simulink model "NDI_model"  (R2021b)
settings: Solver=ode4  StartTime=0.0  StopTime=20  FixedStep=.005  RelTol=1e-3
values from neighbouring files (symbols this model uses):
  A = [0 1; -wn^2 -2*zeta*wn]    [SetupModel.m]
  B = [0;wn^2]    [SetupModel.m]
  C = [eye(2);-wn^2 -2*zeta*wn]    [SetupModel.m]
  D = [0;0;wn^2]    [SetupModel.m]
  dist = 0    [SetupModel.m]
  I = [Ixx 0 -Ixz; 0 Iyy 0; -Ixz 0 Izz]    [NDI_quat.m]    (also in SetupModel.m = [Ixx 0 -Ixz;0 Iyy 0; -Ixz 0 Izz])
  Im = I    [SetupModel.m]
  K = lqr(A,B,Q,R,[])    [SetupModel.m]
  phi = phic(1)    [QuaternionCommand.m]    (also in SetupModel.m = 0.523598775598)
  psi = 45*pi/180    (= 0.785398163397)    [SetupModel.m]
  theta = thetac(1)    [QuaternionCommand.m]    (also in SetupModel.m = -1.0471975512)
  use_error_loop = 0    [SetupModel.m]
  x0 = [0,0,0,1,0,0,0]'    [SetupModel.m]
libraries: matrix_library x2
settings Model: Creator=17165  LastModifiedBy=17165

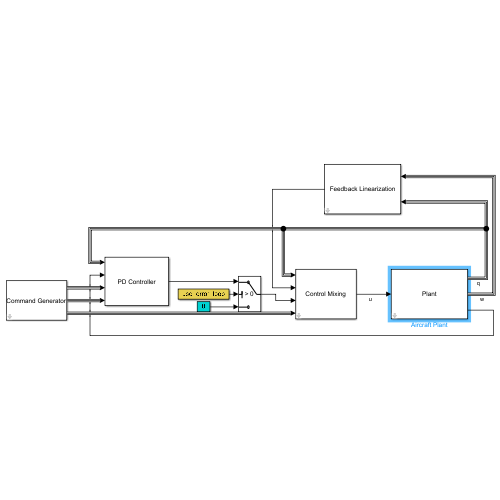
[thumbnail: Simulink's stored preview of the top-level diagram]
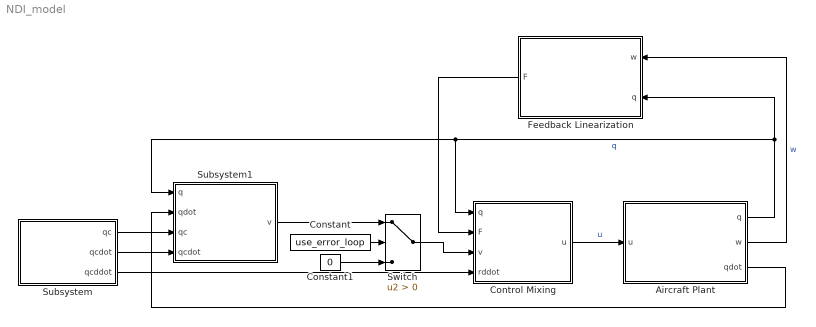
== system NDI_model ==
  Aircraft Plant : Subsystem  mask{I=I, x0=x0, dist=dist}
      mask prompts: I "Plant Moment of Inertia"; x0 "Initial Conditions"; dist "Disturbance Amplitude"
      mask Display: disp('Plant')
  Constant : Constant  Value=use_error_loop
  Constant1 : Constant  Value=0
  Control Mixing : Subsystem  mask{I=Im}
      mask prompts: I "Model Moment of Inertia"
      mask Display: disp('Control Mixing')
  Feedback Linearization : Subsystem  mask{I=Im}
      mask prompts: I "Model Moment of Inertia"
      mask Display: disp('Feedback Linearization')
  Subsystem : Subsystem  mask{A=A, B=B, C=C, D=D, phic=phi, thetac=theta, psic=psi}
      mask prompts: A "Filter A"; B "FIlter B"; C "FIlter C"; D "Filter C"; phic "Roll command"; thetac "Pitch command"; psic "Roll command"
      mask Display: disp('Command Generator')
  Subsystem1 : Subsystem
      mask Display: disp('PD Controller')
  Switch : Switch  Criteria=u2 > Threshold
  wires:
  Aircraft Plant/2(w) -> Feedback Linearization/1(w)  "w"
  Aircraft Plant/1(q) -> Feedback Linearization/2(q), Subsystem1/1(q), Control Mixing/1(q)  "q"
  Control Mixing/1(u) -> Aircraft Plant/1(u)  "u"
  Feedback Linearization/1(F) -> Control Mixing/2(F)
  Subsystem/3(qcddot) -> Control Mixing/4(rddot)
  Subsystem/1(qc) -> Subsystem1/3(qc)
  Subsystem/2(qcdot) -> Subsystem1/4(qcdot)
  Aircraft Plant/3(qdot) -> Subsystem1/2(qdot)
  Switch/1 -> Control Mixing/3(v)
  Subsystem1/1(v) -> Switch/1
  Constant/1 -> Switch/2
  Constant1/1 -> Switch/3

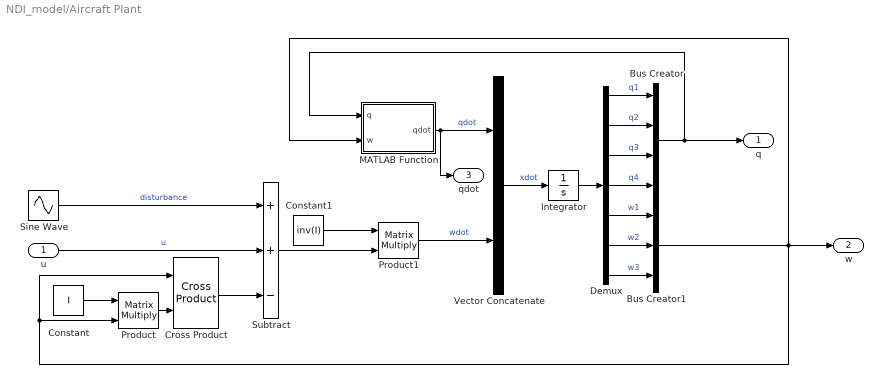
== system NDI_model/Aircraft Plant ==
  u : Inport
  Bus Creator : BusCreator  Inputs=4
  Bus Creator1 : BusCreator  Inputs=3
  Constant : Constant  Value=I
  Constant1 : Constant  Value=inv(I)
  Cross Product : matrix_library/Cross Product
      settings: SourceProductBaseCode=SL
  Demux : Demux  Outputs=7
  Integrator : Integrator  InitialCondition=x0
  MATLAB Function : MATLAB Function  TreatAsAtomicUnit=on
  Product : Product  Multiplication=Matrix(*)
  Product1 : Product  Multiplication=Matrix(*)
  Sine Wave : Sin  Amplitude=dist  SampleTime=0
  Subtract : Sum  Inputs=++-
  Vector Concatenate : Concatenate
  q : Outport
  w : Outport  Port=2
  qdot : Outport  Port=3
  wires:
  Product/1 -> Cross Product/2
  Constant/1 -> Product/1
  Subtract/1 -> Product1/2
  Constant1/1 -> Product1/1
  Product1/1 -> Vector Concatenate/2  "wdot"
  MATLAB Function/1(qdot) -> qdot/1, Vector Concatenate/1  "qdot"
  Vector Concatenate/1 -> Integrator/1  "xdot"
  Integrator/1 -> Demux/1
  Demux/1 -> Bus Creator/1  "q1"
  Demux/4 -> Bus Creator/4  "q4"
  Demux/3 -> Bus Creator/3  "q3"
  Demux/2 -> Bus Creator/2  "q2"
  Demux/5 -> Bus Creator1/1  "w1"
  Demux/6 -> Bus Creator1/2  "w2"
  Demux/7 -> Bus Creator1/3  "w3"
  Bus Creator/1 -> MATLAB Function/1(q), q/1
  Bus Creator1/1 -> w/1, MATLAB Function/2(w), Cross Product/1, Product/2
  Cross Product/1 -> Subtract/3
  u/1 -> Subtract/2  "u"
  Sine Wave/1 -> Subtract/1  "disturbance"

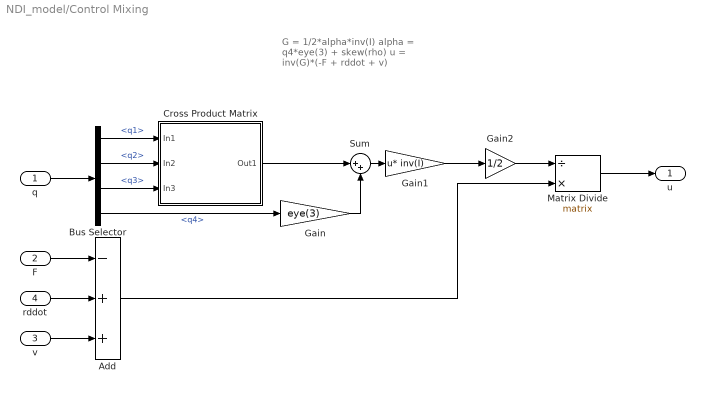
== system NDI_model/Control Mixing ==
  note: G = 1/2*alpha*inv(I)
      |
      | alpha = q4*eye(3) + skew(rho)
      |
      | u = inv(G)*(-F + rddot + v)
  q : Inport
  F : Inport  Port=2
  v : Inport  Port=3
  rddot : Inport  Port=4
  Add : Sum  Inputs=-++
  Bus Selector : BusSelector  OutputSignals=q1,q2,q3,q4
  Cross Product Matrix : Subsystem
      mask Display: disp('Cross Product Matrix')
  Gain : Gain  Gain=eye(3)
  Gain1 : Gain  Gain=inv(I)  Multiplication=Matrix(u*K)
  Gain2 : Gain  Gain=1/2
  Matrix Divide : Product  Inputs=/*  Multiplication=Matrix(*)
  Sum : Sum  Inputs=|++
  u : Outport
  wires:
  F/1 -> Add/1
  rddot/1 -> Add/2
  v/1 -> Add/3
  q/1 -> Bus Selector/1
  Bus Selector/1 -> Cross Product Matrix/1(In1)  "<q1>"
  Bus Selector/2 -> Cross Product Matrix/2(In2)  "<q2>"
  Bus Selector/3 -> Cross Product Matrix/3(In3)  "<q3>"
  Cross Product Matrix/1(Out1) -> Sum/1
  Bus Selector/4 -> Gain/1  "<q4>"
  Gain/1 -> Sum/2
  Sum/1 -> Gain1/1
  Gain1/1 -> Gain2/1
  Gain2/1 -> Matrix Divide/1
  Add/1 -> Matrix Divide/2
  Matrix Divide/1 -> u/1

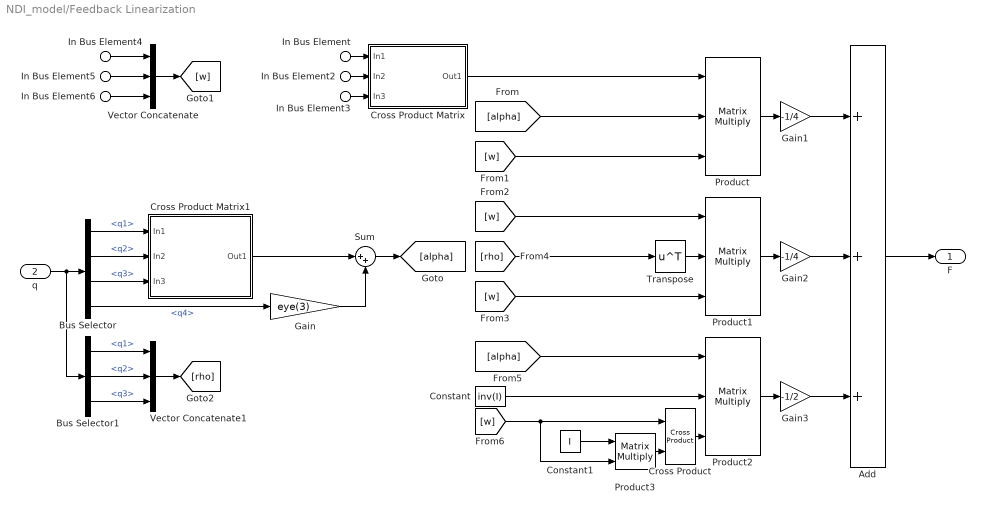
== system NDI_model/Feedback Linearization ==
  In Bus Element : Inport  PortName=w  Element=w1
  In Bus Element4 : Inport  PortName=w  Element=w1
  In Bus Element2 : Inport  PortName=w  Element=w2
  In Bus Element5 : Inport  PortName=w  Element=w2
  In Bus Element3 : Inport  PortName=w  Element=w3
  In Bus Element6 : Inport  PortName=w  Element=w3
  q : Inport  Port=2
  Add : Sum  Inputs=+++
  Bus Selector : BusSelector  OutputSignals=q1,q2,q3,q4
  Bus Selector1 : BusSelector  OutputSignals=q1,q2,q3
  Constant : Constant  Value=inv(I)
  Constant1 : Constant  Value=I
  Cross Product : matrix_library/Cross Product
      settings: SourceProductBaseCode=SL
  Cross Product Matrix : Subsystem
      mask Display: disp('Cross Product Matrix')
  Cross Product Matrix1 : Subsystem
      mask Display: disp('Cross Product Matrix')
  Gain : Gain  Gain=eye(3)
  Gain1 : Gain  Gain=-1/4
  Gain2 : Gain  Gain=-1/4
  Gain3 : Gain  Gain=-1/2
  Product : Product  Inputs=3  Multiplication=Matrix(*)
  Product1 : Product  Inputs=3  Multiplication=Matrix(*)
  Product2 : Product  Inputs=3  Multiplication=Matrix(*)
  Product3 : Product  Multiplication=Matrix(*)
  Sum : Sum  Inputs=|++
  Transpose : Math  Operator=transpose  SaturateOnIntegerOverflow=on
  Vector Concatenate : Concatenate  NumInputs=3
  Vector Concatenate1 : Concatenate  NumInputs=3
  F : Outport
  wires:
  In Bus Element/1 -> Cross Product Matrix/1(In1)
  In Bus Element2/1 -> Cross Product Matrix/2(In2)
  In Bus Element3/1 -> Cross Product Matrix/3(In3)
  In Bus Element5/1 -> Vector Concatenate/2
  In Bus Element4/1 -> Vector Concatenate/1
  In Bus Element6/1 -> Vector Concatenate/3
  Gain/1 -> Sum/2
  Bus Selector/1 -> Cross Product Matrix1/1(In1)  "<q1>"
  Bus Selector/2 -> Cross Product Matrix1/2(In2)  "<q2>"
  q/1 -> Bus Selector1/1, Bus Selector/1
  Cross Product Matrix1/1(Out1) -> Sum/1
  Bus Selector/4 -> Gain/1  "<q4>"
  Bus Selector/3 -> Cross Product Matrix1/3(In3)  "<q3>"
  Sum/1 -> [alpha]
  Cross Product Matrix/1(Out1) -> Product/1
  [alpha] -> Product/2
  Vector Concatenate/1 -> [w]
  [w] -> Product/3
  Bus Selector1/3 -> Vector Concatenate1/3  "<q3>"
  Bus Selector1/1 -> Vector Concatenate1/1  "<q1>"
  Bus Selector1/2 -> Vector Concatenate1/2  "<q2>"
  Vector Concatenate1/1 -> [rho]
  Product/1 -> Gain1/1
  [w] -> Product1/1
  [w] -> Product1/3
  Transpose/1 -> Product1/2
  [rho] -> Transpose/1
  Product1/1 -> Gain2/1
  [alpha] -> Product2/1
  Constant/1 -> Product2/2
  Constant1/1 -> Product3/1
  Product3/1 -> Cross Product/2
  Cross Product/1 -> Product2/3
  [w] -> Product3/2, Cross Product/1
  Product2/1 -> Gain3/1
  Gain2/1 -> Add/2
  Gain1/1 -> Add/1
  Gain3/1 -> Add/3
  Add/1 -> F/1

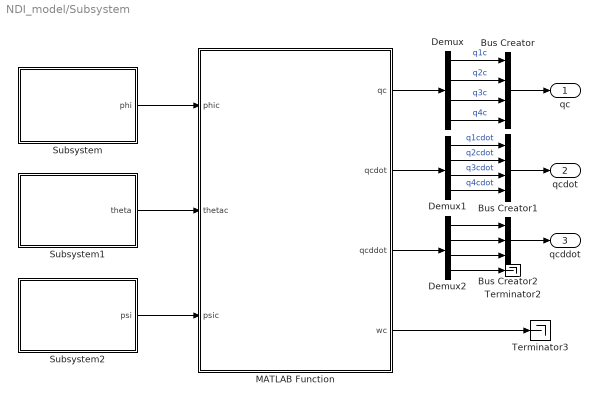
== system NDI_model/Subsystem ==
  Bus Creator : BusCreator  Inputs=4
  Bus Creator1 : BusCreator  Inputs=4
  Bus Creator2 : BusCreator  Inputs=3
  Demux : Demux
  Demux1 : Demux
  Demux2 : Demux
  MATLAB Function : MATLAB Function  TreatAsAtomicUnit=on
  Subsystem : Subsystem  mask{A=A, B=B, C=C, D=D, amp=phic}
      mask prompts: A "FIlter A Matrix"; B "Filter B Matrix"; C "Filter C Matrix"; D "Filter D Matrix"; amp "Quaternion Command"
      mask Display: disp('Filtered Command')
  Subsystem1 : Subsystem  mask{A=A, B=B, C=C, D=D, amp=thetac}
      mask prompts: A "FIlter A Matrix"; B "Filter B Matrix"; C "Filter C Matrix"; D "Filter D Matrix"; amp "Quaternion Command"
      mask Display: disp('Filtered Command')
  Subsystem2 : Subsystem  mask{A=A, B=B, C=C, D=D, amp=psic}
      mask prompts: A "FIlter A Matrix"; B "Filter B Matrix"; C "Filter C Matrix"; D "Filter D Matrix"; amp "Quaternion Command"
      mask Display: disp('Filtered Command')
  Terminator2 : Terminator
  Terminator3 : Terminator
  qc : Outport
  qcdot : Outport  Port=2
  qcddot : Outport  Port=3
  wires:
  Subsystem/1(phi) -> MATLAB Function/1(phic)
  Subsystem1/1(theta) -> MATLAB Function/2(thetac)
  Subsystem2/1(psi) -> MATLAB Function/3(psic)
  MATLAB Function/2(qcdot) -> Demux1/1
  MATLAB Function/1(qc) -> Demux/1
  MATLAB Function/4(wc) -> Terminator3/1
  Demux/4 -> Bus Creator/4  "q4c"
  Bus Creator/1 -> qc/1
  Demux1/2 -> Bus Creator1/2  "q2cdot"
  Bus Creator1/1 -> qcdot/1
  Demux1/1 -> Bus Creator1/1  "q1cdot"
  Demux1/3 -> Bus Creator1/3  "q3cdot"
  Demux1/4 -> Bus Creator1/4  "q4cdot"
  Bus Creator2/1 -> qcddot/1
  MATLAB Function/3(qcddot) -> Demux2/1
  Demux2/1 -> Bus Creator2/1
  Demux2/2 -> Bus Creator2/2
  Demux2/3 -> Bus Creator2/3
  Demux2/4 -> Terminator2/1
  Demux/1 -> Bus Creator/1  "q1c"
  Demux/2 -> Bus Creator/2  "q2c"
  Demux/3 -> Bus Creator/3  "q3c"

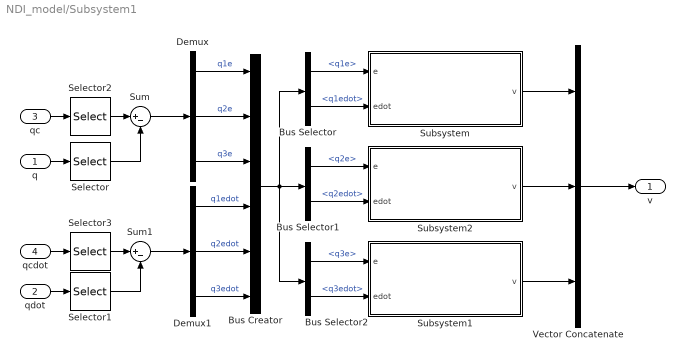
== system NDI_model/Subsystem1 ==
  q : Inport
  qdot : Inport  Port=2
  qc : Inport  Port=3
  qcdot : Inport  Port=4
  Bus Creator : BusCreator  Inputs=6
  Bus Selector : BusSelector  OutputSignals=q1e,q1edot
  Bus Selector1 : BusSelector  OutputSignals=q2e,q2edot
  Bus Selector2 : BusSelector  OutputSignals=q3e,q3edot
  Demux : Demux  Outputs=3
  Demux1 : Demux  Outputs=3
  Selector{,1..3} (4 alike) : Selector  InputPortWidth=4  IndexOptions=Index vector (dialog)  Indices=[1 2 3]  OutputSizes=1
  Subsystem : Subsystem  mask{Kp=K(1), Kd=K(2)}
      mask Display: disp('PD-Compensator')
  Subsystem1 : Subsystem  mask{Kp=K(1), Kd=K(2)}
      mask Display: disp('PD-Compensator')
  Subsystem2 : Subsystem  mask{Kp=K(1), Kd=K(2)}
      mask Display: disp('PD-Compensator')
  Sum : Sum  Inputs=|+-
  Sum1 : Sum  Inputs=|+-
  Vector Concatenate : Concatenate  NumInputs=3
  v : Outport
  wires:
  Vector Concatenate/1 -> v/1
  Subsystem/1(v) -> Vector Concatenate/1
  Subsystem2/1(v) -> Vector Concatenate/2
  Subsystem1/1(v) -> Vector Concatenate/3
  Sum/1 -> Demux/1
  Sum1/1 -> Demux1/1
  Demux/1 -> Bus Creator/1  "q1e"
  Demux/2 -> Bus Creator/2  "q2e"
  Demux/3 -> Bus Creator/3  "q3e"
  Demux1/1 -> Bus Creator/4  "q1edot"
  Demux1/2 -> Bus Creator/5  "q2edot"
  Demux1/3 -> Bus Creator/6  "q3edot"
  Bus Selector/1 -> Subsystem/1(e)  "<q1e>"
  Bus Selector/2 -> Subsystem/2(edot)  "<q1edot>"
  Bus Selector2/2 -> Subsystem1/2(edot)  "<q3edot>"
  Bus Selector2/1 -> Subsystem1/1(e)  "<q3e>"
  Bus Selector1/1 -> Subsystem2/1(e)  "<q2e>"
  Bus Selector1/2 -> Subsystem2/2(edot)  "<q2edot>"
  Bus Creator/1 -> Bus Selector2/1, Bus Selector/1, Bus Selector1/1
  q/1 -> Selector/1
  Selector/1 -> Sum/2
  qdot/1 -> Selector1/1
  Selector1/1 -> Sum1/2
  qc/1 -> Selector2/1
  Selector2/1 -> Sum/1
  qcdot/1 -> Selector3/1
  Selector3/1 -> Sum1/1

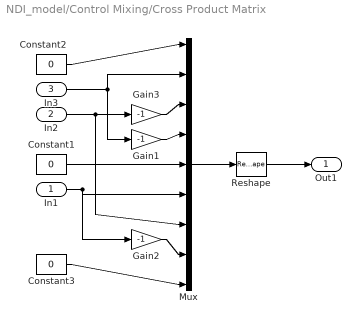
== system NDI_model/Control Mixing/Cross Product Matrix ==
  In1 : Inport
  In2 : Inport  Port=2
  In3 : Inport  Port=3
  Constant1 : Constant  Value=0
  Constant2 : Constant  Value=0
  Constant3 : Constant  Value=0
  Gain1 : Gain  Gain=-1
  Gain2 : Gain  Gain=-1
  Gain3 : Gain  Gain=-1
  Mux : Mux  Inputs=9
  Reshape : Reshape  OutputDimensionality=Customize  OutputDimensions=[3,3]
  Out1 : Outport
  wires:
  Constant2/1 -> Mux/1
  Constant1/1 -> Mux/5
  In1/1 -> Gain2/1, Mux/6
  In3/1 -> Gain1/1, Mux/2
  Constant3/1 -> Mux/9
  Reshape/1 -> Out1/1
  Mux/1 -> Reshape/1
  Gain3/1 -> Mux/3
  In2/1 -> Mux/7, Gain3/1
  Gain1/1 -> Mux/4
  Gain2/1 -> Mux/8

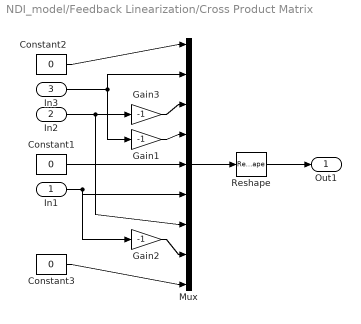
== system NDI_model/Feedback Linearization/Cross Product Matrix ==
  In1 : Inport
  In2 : Inport  Port=2
  In3 : Inport  Port=3
  Constant1 : Constant  Value=0
  Constant2 : Constant  Value=0
  Constant3 : Constant  Value=0
  Gain1 : Gain  Gain=-1
  Gain2 : Gain  Gain=-1
  Gain3 : Gain  Gain=-1
  Mux : Mux  Inputs=9
  Reshape : Reshape  OutputDimensionality=Customize  OutputDimensions=[3,3]
  Out1 : Outport
  wires:
  Constant2/1 -> Mux/1
  Constant1/1 -> Mux/5
  In1/1 -> Gain2/1, Mux/6
  In3/1 -> Gain1/1, Mux/2
  Constant3/1 -> Mux/9
  Reshape/1 -> Out1/1
  Mux/1 -> Reshape/1
  Gain3/1 -> Mux/3
  In2/1 -> Mux/7, Gain3/1
  Gain1/1 -> Mux/4
  Gain2/1 -> Mux/8

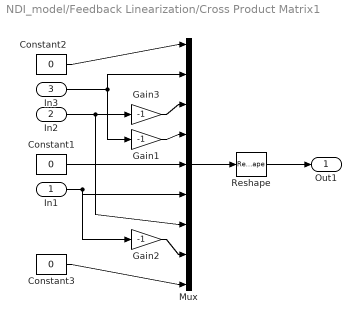
== system NDI_model/Feedback Linearization/Cross Product Matrix1 ==
  In1 : Inport
  In2 : Inport  Port=2
  In3 : Inport  Port=3
  Constant1 : Constant  Value=0
  Constant2 : Constant  Value=0
  Constant3 : Constant  Value=0
  Gain1 : Gain  Gain=-1
  Gain2 : Gain  Gain=-1
  Gain3 : Gain  Gain=-1
  Mux : Mux  Inputs=9
  Reshape : Reshape  OutputDimensionality=Customize  OutputDimensions=[3,3]
  Out1 : Outport
  wires:
  Constant2/1 -> Mux/1
  Constant1/1 -> Mux/5
  In1/1 -> Gain2/1, Mux/6
  In3/1 -> Gain1/1, Mux/2
  Constant3/1 -> Mux/9
  Reshape/1 -> Out1/1
  Mux/1 -> Reshape/1
  Gain3/1 -> Mux/3
  In2/1 -> Mux/7, Gain3/1
  Gain1/1 -> Mux/4
  Gain2/1 -> Mux/8

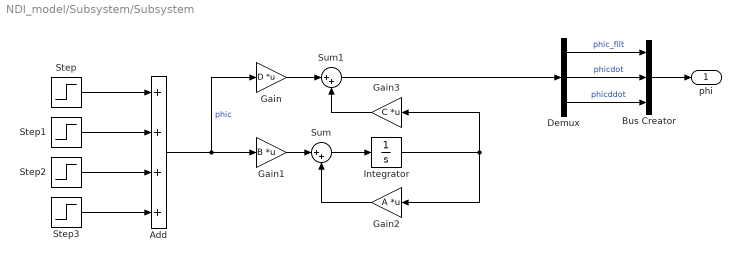
== system NDI_model/Subsystem/Subsystem ==
  Add : Sum  Inputs=++++
  Bus Creator : BusCreator  Inputs=3
  Demux : Demux  Outputs=3
  Gain : Gain  Gain=D  Multiplication=Matrix(K*u)
  Gain1 : Gain  Gain=B  Multiplication=Matrix(K*u)
  Gain2 : Gain  Gain=A  Multiplication=Matrix(K*u)
  Gain3 : Gain  Gain=C  Multiplication=Matrix(K*u)
  Integrator : Integrator
  Step : Step  After=amp  SampleTime=0
  Step1 : Step  Time=6  After=-amp  SampleTime=0
  Step2 : Step  Time=6  After=-amp  SampleTime=0
  Step3 : Step  Time=11  After=amp  SampleTime=0
  Sum : Sum  Inputs=|++
  Sum1 : Sum  Inputs=|++
  phi : Outport
  wires:
  Gain/1 -> Sum1/1
  Sum1/1 -> Demux/1
  Add/1 -> Gain/1, Gain1/1  "phic"
  Step2/1 -> Add/3
  Gain1/1 -> Sum/1
  Integrator/1 -> Gain2/1, Gain3/1
  Step1/1 -> Add/2
  Step/1 -> Add/1
  Gain3/1 -> Sum1/2
  Step3/1 -> Add/4
  Gain2/1 -> Sum/2
  Sum/1 -> Integrator/1
  Bus Creator/1 -> phi/1
  Demux/1 -> Bus Creator/1  "phic_filt"
  Demux/2 -> Bus Creator/2  "phicdot"
  Demux/3 -> Bus Creator/3  "phicddot"

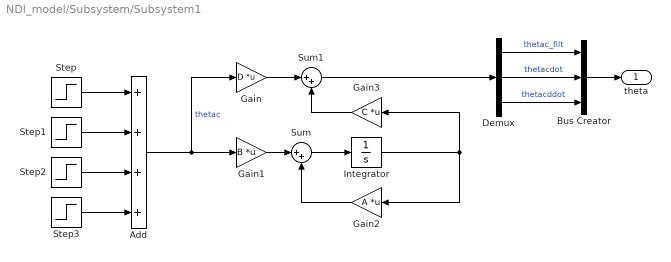
== system NDI_model/Subsystem/Subsystem1 ==
  Add : Sum  Inputs=++++
  Bus Creator : BusCreator  Inputs=3
  Demux : Demux  Outputs=3
  Gain : Gain  Gain=D  Multiplication=Matrix(K*u)
  Gain1 : Gain  Gain=B  Multiplication=Matrix(K*u)
  Gain2 : Gain  Gain=A  Multiplication=Matrix(K*u)
  Gain3 : Gain  Gain=C  Multiplication=Matrix(K*u)
  Integrator : Integrator
  Step : Step  After=amp  SampleTime=0
  Step1 : Step  Time=6  After=-amp  SampleTime=0
  Step2 : Step  Time=6  After=-amp  SampleTime=0
  Step3 : Step  Time=11  After=amp  SampleTime=0
  Sum : Sum  Inputs=|++
  Sum1 : Sum  Inputs=|++
  theta : Outport
  wires:
  Gain/1 -> Sum1/1
  Add/1 -> Gain/1, Gain1/1  "thetac"
  Step2/1 -> Add/3
  Gain1/1 -> Sum/1
  Integrator/1 -> Gain2/1, Gain3/1
  Step1/1 -> Add/2
  Step/1 -> Add/1
  Gain3/1 -> Sum1/2
  Step3/1 -> Add/4
  Gain2/1 -> Sum/2
  Sum/1 -> Integrator/1
  Demux/3 -> Bus Creator/3  "thetacddot"
  Demux/1 -> Bus Creator/1  "thetac_filt"
  Sum1/1 -> Demux/1
  Bus Creator/1 -> theta/1
  Demux/2 -> Bus Creator/2  "thetacdot"

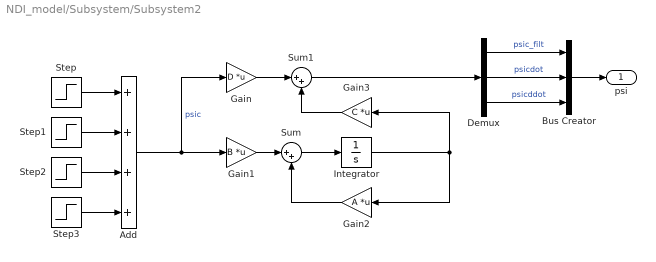
== system NDI_model/Subsystem/Subsystem2 ==
  Add : Sum  Inputs=++++
  Bus Creator : BusCreator  Inputs=3
  Demux : Demux  Outputs=3
  Gain : Gain  Gain=D  Multiplication=Matrix(K*u)
  Gain1 : Gain  Gain=B  Multiplication=Matrix(K*u)
  Gain2 : Gain  Gain=A  Multiplication=Matrix(K*u)
  Gain3 : Gain  Gain=C  Multiplication=Matrix(K*u)
  Integrator : Integrator
  Step : Step  After=amp  SampleTime=0
  Step1 : Step  Time=6  After=-amp  SampleTime=0
  Step2 : Step  Time=6  After=-amp  SampleTime=0
  Step3 : Step  Time=11  After=amp  SampleTime=0
  Sum : Sum  Inputs=|++
  Sum1 : Sum  Inputs=|++
  psi : Outport
  wires:
  Gain/1 -> Sum1/1
  Add/1 -> Gain/1, Gain1/1  "psic"
  Step2/1 -> Add/3
  Gain1/1 -> Sum/1
  Integrator/1 -> Gain2/1, Gain3/1
  Step1/1 -> Add/2
  Step/1 -> Add/1
  Gain3/1 -> Sum1/2
  Step3/1 -> Add/4
  Gain2/1 -> Sum/2
  Sum/1 -> Integrator/1
  Demux/3 -> Bus Creator/3  "psicddot"
  Demux/1 -> Bus Creator/1  "psic_filt"
  Sum1/1 -> Demux/1
  Bus Creator/1 -> psi/1
  Demux/2 -> Bus Creator/2  "psicdot"

== system NDI_model/Subsystem1/Subsystem ==
  e : Inport
  edot : Inport  Port=2
  Gain : Gain  Gain=Kp
  Gain1 : Gain  Gain=Kd
  Sum : Sum  Inputs=|++
  v : Outport
  wires:
  e/1 -> Gain/1
  Gain/1 -> Sum/1
  edot/1 -> Gain1/1
  Gain1/1 -> Sum/2
  Sum/1 -> v/1

== system NDI_model/Subsystem1/Subsystem1 ==
  e : Inport
  edot : Inport  Port=2
  Gain : Gain  Gain=Kp
  Gain1 : Gain  Gain=Kd
  Sum : Sum  Inputs=|++
  v : Outport
  wires:
  e/1 -> Gain/1
  Gain/1 -> Sum/1
  edot/1 -> Gain1/1
  Gain1/1 -> Sum/2
  Sum/1 -> v/1

== system NDI_model/Subsystem1/Subsystem2 ==
  e : Inport
  edot : Inport  Port=2
  Gain : Gain  Gain=Kp
  Gain1 : Gain  Gain=Kd
  Sum : Sum  Inputs=|++
  v : Outport
  wires:
  e/1 -> Gain/1
  Gain/1 -> Sum/1
  edot/1 -> Gain1/1
  Gain1/1 -> Sum/2
  Sum/1 -> v/1

== matlab function NDI_model/Aircraft Plant/MATLAB Function ==
  data: q input; qdot output; w input
function qdot = fcn(q,w)
qdot = QuaternionKinematics([],q,w);

end

== matlab function NDI_model/Subsystem/MATLAB Function ==
  data: phic input; thetac input; psic input; qc output; qcdot output; qcddot output; wc output
function [qc,qcdot, qcddot, wc] = QuaternionCommandGenerator(phic,thetac,psic)
qc      = zeros(4,1);
qcdot   = zeros(4,1);
qcddot  = zeros(4,1);
[qc,qcdot, qcddot, wc] = QuaternionCommand(phic,thetac,psic);


end
